simulink model "MODELO_ROLLOVER"  (R2023a)
settings: Solver=VariableStepAuto  StartTime=0.0  StopTime=5  RelTol=1e-3
values from neighbouring files (symbols this model uses):
  A = E1*F    [CONTROL_ROLL_OVER.m]    (also in Modelo_roll_control.m; State_space_robust.m; calc_KMax1.m; calc_KMax2.m)
  B = E1*G    [CONTROL_ROLL_OVER.m]    (also in Modelo_roll_control.m; State_space_robust.m; calc_KMax1.m; calc_KMax2.m)
  C = eye(4)    [CONTROL_ROLL_OVER.m]    (also in Modelo_roll_control.m; State_space_robust.m)
  D = zeros(4,1)    [CONTROL_ROLL_OVER.m]    (also in Modelo_roll_control.m = zeros(1,4); State_space_robust.m = zeros(1,4))
  k = H_inf_robust(A1,A2,A3,A4,B1,B2,B3,B4,W1,W2,W3,W4,C1,D12,D11)    [CONTROL_ROLL_OVER.m]    (also in Modelo_roll_control.m; State_space_robust.m)
  W = B    [CONTROL_ROLL_OVER.m]    (also in Modelo_roll_control.m; State_space_robust.m; calc_KMax1.m; calc_KMax2.m)
undefined symbols (not defined in the file or in its folder): sigbuilder_block
settings Model: Creator=csanc  LastModifiedBy=csanc

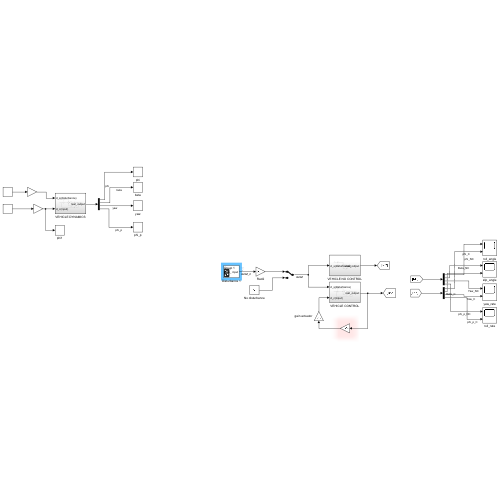
[thumbnail: Simulink's stored preview of the top-level diagram]
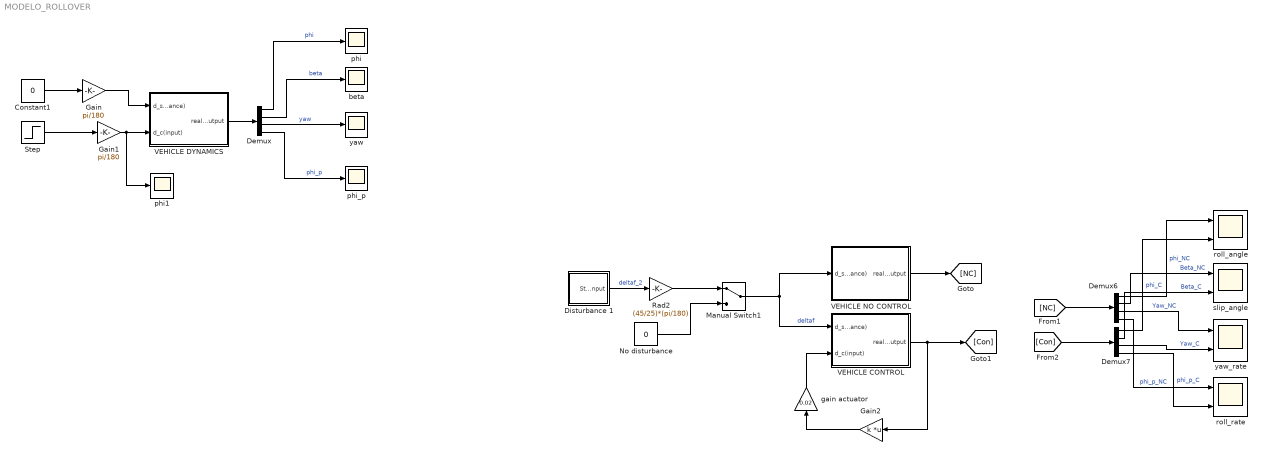
== system MODELO_ROLLOVER ==
  Constant1 : Constant  Value=0
  Demux : Demux
  Demux6 : Demux
  Demux7 : Demux
  Disturbance 1 : Subsystem  Tag=STV Subsys  LoadFcn=sigbuilder_block('load');  StartFcn=sigbuilder_block('start');  StopFcn=sigbuilder_block('stop');  ClipboardFcn=sigbuilder_block('clipboard');  mask(Sigbuilder block){tuvar=[0:10]}
      mask help: Simulink:masks:SigbuilderBlock_MD
      mask init:
      | if ~strcmp(get_param(bdroot(gcbh),'SimulationStatus'),'stopped') tuvar = sigbuilder_block('maskInit'); end
      settings: CopyFcn=sigbuilder_block('copy');  DeleteFcn=sigbuilder_block('delete');  ModelCloseFcn=sigbuilder_block('modelClose');  PreSaveFcn=sigbuilder_block('preSave');  PauseFcn=sigbuilder_block('pause');  ContinueFcn=sigbuilder_block('continue');  NameChangeFcn=sigbuilder_block('namechange');  OpenFcn=sigbuilder_block('open',[265.8 141.6 550.8 400.2 ]);  CloseFcn=sigbuilder_block('close');
      mask Display: plot(0, 0, 100, 100,[2, 2, 32, 32, 2], [68, 8, 8, 68, 68],[32, 2], [38, 38], [32, 19, 2],[53, 60, 44], [32, 17, 17, 2],[16, 16, 31, 31]);txt = getActiveGroup(gcbh);text(2, 100, txt,'verticalAlignment', 'top');
  Gain : Gain  Gain=pi/180
  Gain1 : Gain  Gain=pi/180
  Gain2 : Gain  Gain=k  Multiplication=Matrix(K*u)
  Manual Switch1 : ManualSwitch
  No disturbance : Constant  Value=0
  Rad2 : Gain  Gain=(45/25)*(pi/180)
  Step : Step  Time=0  After=3  SampleTime=0
  VEHICLE CONTROL : Subsystem
  VEHICLE DYNAMICS : Subsystem
  VEHICLE NO CONTROL : Subsystem
  beta : Scope
  gain actuator : Gain  Gain=0.02
  phi : Scope
  phi1 : Scope
  phi_p : Scope
  roll_angle : Scope  NumInputPorts=2
  roll_rate : Scope  NumInputPorts=2
  slip_angle : Scope  NumInputPorts=2
  yaw : Scope
  yaw_rate : Scope  NumInputPorts=2
  wires:
  VEHICLE DYNAMICS/1(real_output) -> Demux/1
  Demux/1 -> phi/1  "phi"
  Demux/2 -> beta/1  "beta"
  Demux/3 -> yaw/1  "yaw"
  Demux/4 -> phi_p/1  "phi_p"
  Gain/1 -> VEHICLE DYNAMICS/1(d_s(disturbance))
  Constant1/1 -> Gain/1
  Step/1 -> Gain1/1
  Gain1/1 -> phi1/1, VEHICLE DYNAMICS/2(d_c(input))
  Manual Switch1/1 -> VEHICLE CONTROL/1(d_s(disturbance)), VEHICLE NO CONTROL/1(d_s(disturbance))  "deltaf"
  VEHICLE NO CONTROL/1(real_output) -> [NC]
  VEHICLE CONTROL/1(real_output) -> Gain2/1, [Con]
  [Con] -> Demux7/1
  [NC] -> Demux6/1
  No disturbance/1 -> Manual Switch1/2
  Demux6/1 -> roll_angle/1  "phi_NC"
  Demux7/1 -> roll_angle/2  "phi_C"
  Demux6/2 -> slip_angle/1  "Beta_NC"
  Demux6/3 -> yaw_rate/1  "Yaw_NC"
  Demux7/3 -> yaw_rate/2  "Yaw_C"
  Demux6/4 -> roll_rate/1  "phi_p_NC"
  Demux7/4 -> roll_rate/2  "phi_p_C"
  Demux7/2 -> slip_angle/2  "Beta_C"
  Disturbance 1/1(Steering angle_ input) -> Rad2/1  "deltaf_2"
  Gain2/1 -> gain actuator/1
  gain actuator/1 -> VEHICLE CONTROL/2(d_c(input))
  Rad2/1 -> Manual Switch1/1

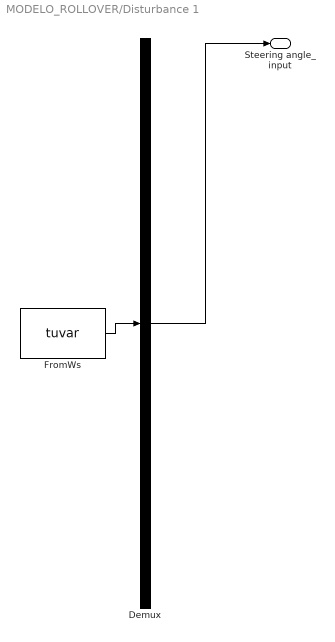
== system MODELO_ROLLOVER/Disturbance 1 ==
  Demux : Demux  Tag=STV Demux  Outputs=1
      settings: DisplayOption=none
  FromWs : FromWorkspace  Tag=STV FromWs  VariableName=tuvar
      SigBuilderData=|
      | common.afterFinalStr = 'Extrapolate'
      | common.sampleTime = 0
      | dataSet.timeRange = [0 3]
      | dataSet.name = 'Group 1'
      | sbobj.Groups.Name = 'Group 1'
      | sbobj.Groups.Signals.Name = 'Steering angle_ input'
      | sbobj.Groups.Signals.XData = [0 0.187490625469 0.374981250937 0.562471876406 0.749962501875 0.937453127344 1.12494375281 1.31243437828 1.49992500375 1.68741562922 1.87490625469 2.06239688016 2.24988750562 2.43737813109 2.62486875656 2.81235938203 2.9998500075 3]
      | sbobj.Groups.Signals.YData = [0 0.565685424949 0.8 0.565685424949 9.79717439318e-17 -0.565685424949 -0.8 -0.565685424949 0 0 0 0 0 0 0 0 0 0]
      | sbobj.Groups.TimeRange = [0 3]
  Steering angle_ input : Outport  Tag=STV Outport
  wires:
  FromWs/1 -> Demux/1
  Demux/1 -> Steering angle_ input/1

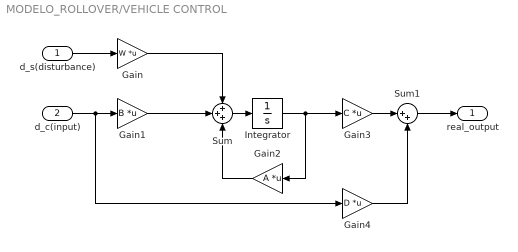
== system MODELO_ROLLOVER/VEHICLE CONTROL ==
  d_s(disturbance) : Inport
  d_c(input) : Inport  Port=2
  Gain : Gain  Gain=W  Multiplication=Matrix(K*u)
  Gain1 : Gain  Gain=B  Multiplication=Matrix(K*u)
  Gain2 : Gain  Gain=A  Multiplication=Matrix(K*u)
  Gain3 : Gain  Gain=C  Multiplication=Matrix(K*u)
  Gain4 : Gain  Gain=D  Multiplication=Matrix(K*u)
  Integrator : Integrator  InitialCondition=[0, 0, 0, 0]
  Sum : Sum  Inputs=+++
  Sum1 : Sum  Inputs=|++
  real_output : Outport
  wires:
  Gain1/1 -> Sum/2
  Gain4/1 -> Sum1/2
  d_s(disturbance)/1 -> Gain/1
  Integrator/1 -> Gain3/1, Gain2/1
  Gain/1 -> Sum/1
  Sum1/1 -> real_output/1
  Gain3/1 -> Sum1/1
  Sum/1 -> Integrator/1
  Gain2/1 -> Sum/3
  d_c(input)/1 -> Gain4/1, Gain1/1

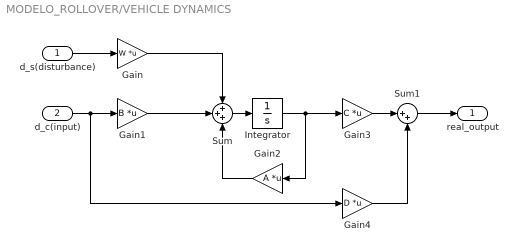
== system MODELO_ROLLOVER/VEHICLE DYNAMICS ==
  d_s(disturbance) : Inport
  d_c(input) : Inport  Port=2
  Gain : Gain  Gain=W  Multiplication=Matrix(K*u)
  Gain1 : Gain  Gain=B  Multiplication=Matrix(K*u)
  Gain2 : Gain  Gain=A  Multiplication=Matrix(K*u)
  Gain3 : Gain  Gain=C  Multiplication=Matrix(K*u)
  Gain4 : Gain  Gain=D  Multiplication=Matrix(K*u)
  Integrator : Integrator  InitialCondition=[0, 0, 0, 0]
  Sum : Sum  Inputs=+++
  Sum1 : Sum  Inputs=|++
  real_output : Outport
  wires:
  Gain1/1 -> Sum/2
  Gain4/1 -> Sum1/2
  d_s(disturbance)/1 -> Gain/1
  Integrator/1 -> Gain3/1, Gain2/1
  Gain/1 -> Sum/1
  Sum1/1 -> real_output/1
  Gain3/1 -> Sum1/1
  Sum/1 -> Integrator/1
  Gain2/1 -> Sum/3
  d_c(input)/1 -> Gain4/1, Gain1/1

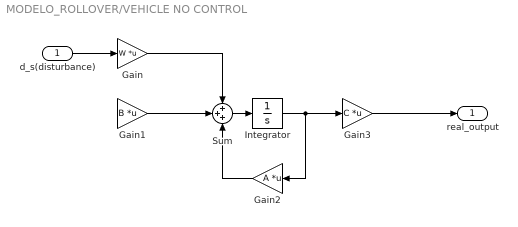
== system MODELO_ROLLOVER/VEHICLE NO CONTROL ==
  d_s(disturbance) : Inport
  Gain : Gain  Gain=W  Multiplication=Matrix(K*u)
  Gain1 : Gain  Gain=B  Multiplication=Matrix(K*u)
  Gain2 : Gain  Gain=A  Multiplication=Matrix(K*u)
  Gain3 : Gain  Gain=C  Multiplication=Matrix(K*u)
  Integrator : Integrator  InitialCondition=[0, 0, 0, 0]
  Sum : Sum  Inputs=+++
  real_output : Outport
  wires:
  Gain1/1 -> Sum/2
  d_s(disturbance)/1 -> Gain/1
  Integrator/1 -> Gain3/1, Gain2/1
  Gain/1 -> Sum/1
  Gain3/1 -> real_output/1
  Sum/1 -> Integrator/1
  Gain2/1 -> Sum/3
